simulink model "V511_L4_TDI"  (R2023b)
settings: Solver=VariableStepAuto  StartTime=0.0  StopTime=110  MaxStep=0.01  RelTol=1e-3
settings Model: Creator=td  LastModifiedBy=killer
settings SolverCC: AlgebraicLoopSolver=TrustRegion
settings DataIOCC: ReturnWorkspaceOutputs=off
settings DebuggingCC: UnconnectedInputMsg=warning  UnconnectedOutputMsg=warning  UnconnectedLineMsg=warning  ArithmeticOperatorsInVariantConditions=warning
settings ModelReferenceCC: EnableRefExpFcnMdlSchedulingChecks=on
settings SFSimCC: CustomCodeUndefinedFunction=UseInterfaceOnly

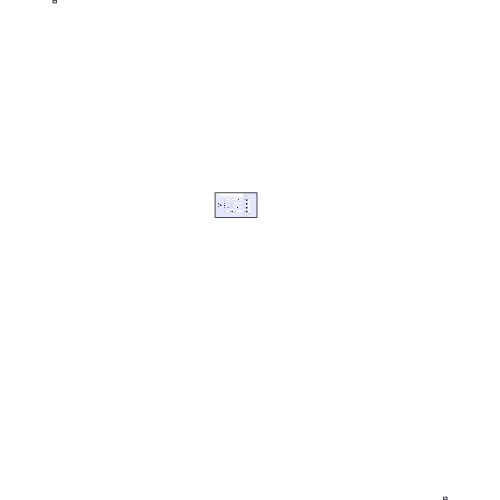
[thumbnail: Simulink's stored preview of the top-level diagram]
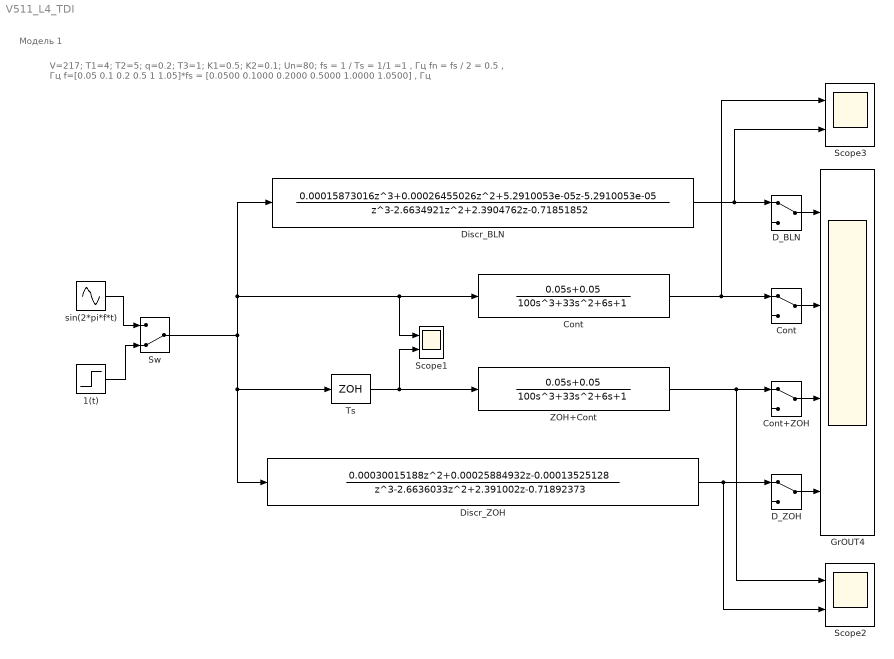
== system V511_L4_TDI ==
  note: Модель 1
  note: V=217; T1=4; T2=5; q=0.2; T3=1; K1=0.5; K2=0.1; Un=80;
      |
      | fs = 1 / Ts = 1/1 =1 , Гц
      | fn = fs / 2 = 0.5 , Гц
      |
      | f=[0.05 0.1 0.2 0.5 1 1.05]*fs = [0.0500 0.1000 0.2000 0.5000 1.0000 1.0500] , Гц
  " Sw  " : ManualSwitch  CurrentSetting=0
  1(t) : Step  Time=0  SampleTime=0
  Cont : TransferFcn  Numerator="[0              0           0.05           0.05]"  Denominator="[ 100             33              6              1 ]"
  "Cont " : ManualSwitch
  "Cont+ZOH " : ManualSwitch
  D_BLN : ManualSwitch
  D_ZOH : ManualSwitch
  Discr_BLN : DiscreteTransferFcn  Numerator="[ 0.00015873016  0.00026455026  5.2910053e-05 -5.2910053e-05 ]"  Denominator="[ 1     -2.6634921      2.3904762    -0.71851852 ]"  SampleTime=0.5
  Discr_ZOH : DiscreteTransferFcn  Numerator="[ 0  0.00030015188  0.00025884932 -0.00013525128 ]"  Denominator="[ 1     -2.6636033       2.391002    -0.71892373 ]"  SampleTime=0.5
  GrOUT4 : Scope  NumInputPorts=4
  Scope1 : Scope  NumInputPorts=2
  Scope2 : Scope  NumInputPorts=2
  Scope3 : Scope  NumInputPorts=2
  Ts : ZeroOrderHold  SampleTime=0.5
  ZOH+Cont : TransferFcn  Numerator="[ 0              0           0.05            0.05 ]"  Denominator="[ 100             33              6              1 ]"
  sin(2*pi*f*t) : Sin  Frequency=2*pi*1.05  SampleTime=0
  wires:
  " Sw  "/1 -> Discr_BLN/1, Cont/1, Scope1/1, Discr_ZOH/1, Ts/1
  Ts/1 -> ZOH+Cont/1, Scope1/2
  Cont/1 -> "Cont "/1, Scope3/1
  Discr_BLN/1 -> D_BLN/1, Scope3/2
  Discr_ZOH/1 -> Scope2/2, D_ZOH/1
  ZOH+Cont/1 -> Scope2/1, "Cont+ZOH "/1
  D_BLN/1 -> GrOUT4/1
  "Cont "/1 -> GrOUT4/2
  "Cont+ZOH "/1 -> GrOUT4/3
  D_ZOH/1 -> GrOUT4/4
  sin(2*pi*f*t)/1 -> " Sw  "/1
  1(t)/1 -> " Sw  "/2
